simulink model "sampleModel26"  (Simulink 9.1)
settings: Solver=VariableStepAuto  StartTime=0.0  StopTime=10.0  RelTol=1e-3
undefined symbols (not defined in the file): DiscIntNeverNeededParam, Newton, Raphson
libraries: simulink x50
(part 1 of 2)
settings Model: Creator=DELL  LastModifiedBy=DELL
settings DataIOCC: SaveFormat=Dataset
settings OptimizationCC: LifeSpan=auto
settings DebuggingCC: UnderspecifiedInitializationDetection=Simplified  MergeDetectMultiDrivingBlocksExec=error  SFUnexpectedBacktrackingDiag=error  SFNoUnconditionalDefaultTransitionDiag=error  SFExecutionAtInitializationDiag=warning
settings HardwareCC: ProdBitPerPointer=64  ProdBitPerSizeT=64  ProdBitPerPtrDiffT=64  ProdLargestAtomicFloat=Float  ProdIntDivRoundTo=Zero  ProdEndianess=LittleEndian  ProdWordSize=64  ProdHWDeviceType=Intel->x86-64 (Windows64)
settings ModelReferenceCC: PropagateSignalLabelsOutOfModel=on
settings CodeAppCC: StateflowObjectComments=off
settings GRTTargetCC: TargetLangStandard=C99 (ISO)  CombineOutputUpdateFcns=on  GRTInterface=off
settings ConfigComp: CovMetricSettings=dwe  CovHtmlReporting=off  CovSaveCumulativeToWorkspaceVar=off  CovSaveSingleToWorkspaceVar=off  CovExternalEMLEnable=on

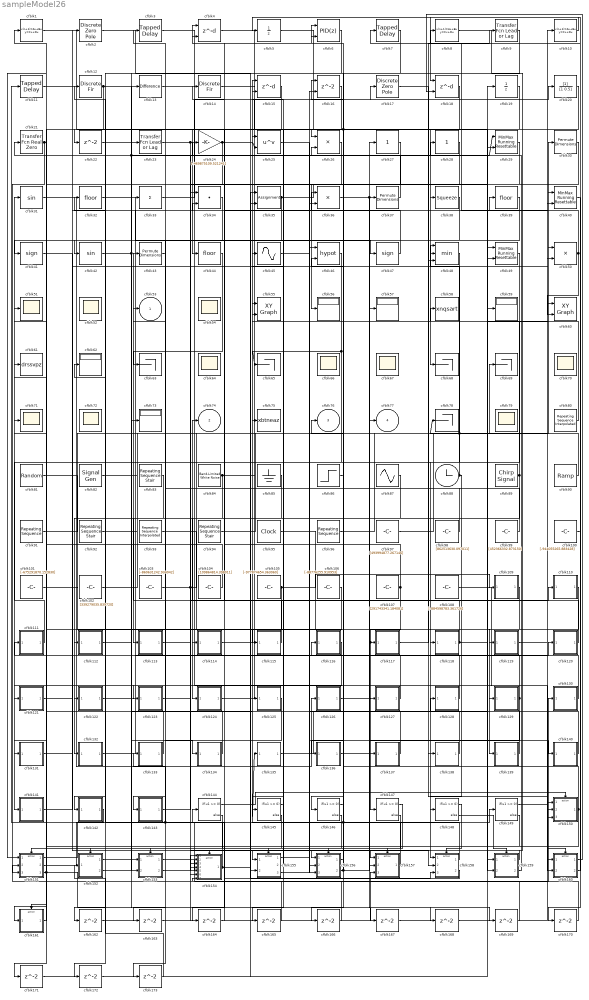
== system sampleModel26 ==
  cfblk1 : DiscreteStateSpace
  cfblk10 : DiscreteStateSpace
  cfblk100 : Constant  Value=[-944055265.883428]  SampleTime=1
  cfblk101 : Constant  Value=[-675291870.152830]  SampleTime=1
  cfblk102 : Constant  Value=[339279035.839720]  SampleTime=1
  cfblk103 : Constant  Value=[-860631242.934042]  SampleTime=1
  cfblk104 : Constant  Value=[109864814.398011]  SampleTime=1
  cfblk105 : Constant  Value=[-977874654.363060]  SampleTime=1
  cfblk106 : Constant  Value=[-88776255.910953]  SampleTime=1
  cfblk107 : Constant  Value=[291743341.184081]  SampleTime=1
  cfblk108 : Constant  Value=[-884598783.361726]  SampleTime=1
  cfblk109 : Subsystem
  cfblk11 : simulink/Discrete/Tapped Delay  vinit=0.0  samptime=-1  NumDelays=1  DelayOrder=Oldest  includeCurrent=off
  cfblk110 : Subsystem
  cfblk111 : Subsystem
  cfblk112 : Subsystem
  cfblk113 : Subsystem
  cfblk114 : Subsystem
  cfblk115 : Subsystem
  cfblk116 : Subsystem
  cfblk117 : Subsystem
  cfblk118 : Subsystem
  cfblk119 : Subsystem
  cfblk12 : DiscreteFir  SampleTime=1
  cfblk120 : Subsystem
  cfblk121 : Subsystem
  cfblk122 : Subsystem
  cfblk123 : Subsystem
  cfblk124 : Subsystem
  cfblk125 : Subsystem
  cfblk126 : Subsystem
  cfblk127 : Subsystem
  cfblk128 : Subsystem
  cfblk129 : Subsystem
  cfblk13 : simulink/Discrete/Difference  ICPrevInput=0.0  OutMin=[]  OutMax=[]  OutDataTypeStr=Inherit: Inherit via back propagation  OutDataType=fixdt(1, 16)  OutScaling=2^-10  DoSatur=off
  cfblk130 : Subsystem
  cfblk131 : Subsystem
  cfblk132 : Subsystem
  cfblk133 : Subsystem
  cfblk134 : Subsystem
  cfblk135 : Subsystem
  cfblk136 : Subsystem
  cfblk137 : Subsystem
  cfblk138 : Subsystem
  cfblk139 : Subsystem
  cfblk14 : DiscreteFir  SampleTime=1
  cfblk140 : Subsystem
  cfblk141 : Subsystem
  cfblk142 : Subsystem
  cfblk143 : Subsystem
  cfblk{144..149} (6 alike) : If  IfExpression=u1 >= 0  SampleTime=1
  cfblk15 : Delay  DelayLengthSource=Input port  SampleTime=1
      settings: InputPortMap=u0,p1
  cfblk150 : Subsystem  TreatAsAtomicUnit=on
  cfblk151 : Subsystem  TreatAsAtomicUnit=on
  cfblk152 : Subsystem  TreatAsAtomicUnit=on
  cfblk153 : Subsystem  TreatAsAtomicUnit=on
  cfblk154 : Subsystem  TreatAsAtomicUnit=on
  cfblk155 : Subsystem  TreatAsAtomicUnit=on
  cfblk156 : Subsystem  TreatAsAtomicUnit=on
  cfblk157 : Subsystem  TreatAsAtomicUnit=on
  cfblk158 : Subsystem  TreatAsAtomicUnit=on
  cfblk159 : Subsystem  TreatAsAtomicUnit=on
  cfblk16 : Delay  ShowEnablePort=on  SampleTime=1
      settings: InputPortMap=u0,e6
  cfblk160 : Subsystem  TreatAsAtomicUnit=on
  cfblk161 : Subsystem  TreatAsAtomicUnit=on
  cfblk{22,162..173} (13 alike) : Delay  SampleTime=1
  cfblk17 : DiscreteZeroPole  Poles=[0 0.5]  Gain=1
  cfblk18 : Delay  DelayLengthSource=Input port  SampleTime=1
      settings: InputPortMap=u0,p1
  cfblk19 : UnitDelay
  cfblk2 : DiscreteZeroPole  Poles=[0 0.5]  Gain=1
  cfblk20 : DiscreteFilter  SampleTime=1
  cfblk21 : simulink/Discrete/Transfer Fcn Real Zero  ZeroZ=0.75  ICPrevInput=0.0  DoSatur=off
      settings: SourceProductName=Simulink  SourceProductBaseCode=SL
  cfblk23 : simulink/Discrete/Transfer Fcn Lead or Lag  PoleZ=0.95  ZeroZ=0.75  ICPrevOutput=0.0  ICPrevInput=0.0  DoSatur=off
      settings: SourceProductName=Simulink  SourceProductBaseCode=SL
  cfblk24 : Gain  Gain=[-469875109.521241]
  cfblk25 : Math  Operator=pow  SaturateOnIntegerOverflow=on
  cfblk26 : Product  Inputs=**
  cfblk27 : simulink/Math Operations/Slider Gain  gain=1  low=0  high=2
  cfblk28 : simulink/Math Operations/Slider Gain  gain=1  low=0  high=2
  cfblk29 : simulink/Math Operations/MinMax Running Resettable  Function=min  vinit=0.0
  cfblk3 : simulink/Discrete/Tapped Delay  vinit=0.0  samptime=-1  NumDelays=1  DelayOrder=Oldest  includeCurrent=off
  cfblk30 : PermuteDimensions
  cfblk31 : Trigonometry
  cfblk32 : Rounding
  cfblk33 : Sum  Inputs=+
  cfblk34 : DotProduct  InputSameDT=on  OutDataTypeStr=Inherit: Inherit via internal rule
  cfblk35 : Assignment  DiagnosticForDimensions=Warning  IndexOptions=Index vector (dialog)  Indices=1  OutputSizes=1
  cfblk36 : Product  Inputs=**
  cfblk37 : PermuteDimensions
  cfblk38 : Squeeze
  cfblk39 : Rounding
  cfblk4 : Delay  DelayLengthSource=Input port  SampleTime=1
      settings: InputPortMap=u0,p1
  cfblk40 : simulink/Math Operations/MinMax Running Resettable  Function=min  vinit=0.0
  cfblk41 : Signum
  cfblk42 : Trigonometry
  cfblk43 : PermuteDimensions
  cfblk44 : Rounding
  cfblk45 : Sin  TimeSource=Use external signal  SampleTime=0
  cfblk46 : Math  Operator=hypot  SaturateOnIntegerOverflow=on
  cfblk47 : Signum
  cfblk48 : MinMax  Inputs=3
  cfblk49 : simulink/Math Operations/MinMax Running Resettable  Function=min  vinit=0.0
  cfblk5 : UnitDelay
  cfblk50 : Product  Inputs=**
  cfblk{51..52,54,64,66..67,70..72,79} (10 alike) : Scope
      cfblk52 settings: Floating=on
      cfblk54 settings: Floating=on
      cfblk64 settings: Floating=on
      cfblk66 settings: Floating=on
      cfblk67 settings: Floating=on
      cfblk70 settings: Floating=on
      cfblk72 settings: Floating=on
      cfblk79 settings: Floating=on
  cfblk55 : simulink/Sinks/XY Graph  xmin=-1  xmax=1  ymin=-1  ymax=1  st=-1
  cfblk{56..57,59,62,73} (5 alike) : Display
  cfblk58 : ToWorkspace  VariableName=xnqsart  SaveFormat=Timeseries  SampleTime=-1
  cfblk6 : simulink/Continuous/PID Controller (2DOF)  Controller=PID  TimeDomain=Discrete-time  SampleTime=1  IntegratorMethod=Forward Euler  FilterMethod=Forward Euler  Form=Parallel  UseFilter=on  ControllerParametersSource=internal  P=1  I=1  D=0  N=100  b=1  c=1  InitialConditionSource=internal  InitialConditionForIntegrator=0  InitialConditionForFilter=0  ExternalReset=none  LimitOutput=off  UpperSaturationLimit=inf  LowerSaturationLimit=-inf  LinearizeAsGain=off  AntiWindupMode=none  Kb=1  TrackingMode=off  Kt=1  PParamMin=[]  PParamMax=[]  IParamMin=[]  IParamMax=[]  DParamMin=[]  DParamMax=[]  NParamMin=[]  NParamMax=[]  bParamMin=[]  bParamMax=[]  cParamMin=[]  cParamMax=[]  KbParamMin=[]  KbParamMax=[]  KtParamMin=[]  KtParamMax=[]  POutMin=[]  POutMax=[]  IOutMin=[]  IOutMax=[]  DOutMin=[]  DOutMax=[]  NOutMin=[]  NOutMax=[]  bOutMin=[]  bOutMax=[]  cOutMin=[]  cOutMax=[]  KbOutMin=[]  KbOutMax=[]  KtOutMin=[]  KtOutMax=[]  IntegratorOutMin=[]  IntegratorOutMax=[]  FilterOutMin=[]  FilterOutMax=[]  SumOutMin=[]  SumOutMax=[]  Sum1OutMin=[]  Sum1OutMax=[]  Sum2OutMin=[]  Sum2OutMax=[]  Sum3OutMin=[]  Sum3OutMax=[]  SumI1OutMin=[]  SumI1OutMax=[]  SumI2OutMin=[]  SumI2OutMax=[]  SumI3OutMin=[]  SumI3OutMax=[]  SumDOutMin=[]  SumDOutMax=[]  SaturationOutMin=[]  SaturationOutMax=[]  IntegratorContinuousStateAttributes=''  IntegratorStateMustResolveToSignalObject=off  IntegratorRTWStateStorageClass=Auto  FilterContinuousStateAttributes=''  FilterStateMustResolveToSignalObject=off  FilterRTWStateStorageClass=Auto  DifferentiatorICPrevScaledInput=0  DifferentiatorOutMin=[]  DifferentiatorOutMax=[]  FilterDiffOutCoefMin=[]  FilterDiffOutCoefMax=[]  SumDenOutMin=[]  SumDenOutMax=[]  SumNumOutMin=[]  SumNumOutMax=[]  ReciprocalOutMin=[]  ReciprocalOutMax=[]  DivideOutMin=[]  DivideOutMax=[]  TunerSelectOption=Transfer Function Based (PID Tuner App)
  cfblk60 : simulink/Sinks/XY Graph  xmin=-1  xmax=1  ymin=-1  ymax=1  st=-1
  cfblk61 : ToWorkspace  VariableName=drssvpz  SaveFormat=Timeseries  SampleTime=-1
  cfblk{63,65,68..69,78} (5 alike) : Terminator
  cfblk7 : simulink/Discrete/Tapped Delay  vinit=0.0  samptime=-1  NumDelays=1  DelayOrder=Oldest  includeCurrent=off
  cfblk75 : ToWorkspace  VariableName=xbtneaz  SaveFormat=Timeseries  SampleTime=-1
  cfblk8 : DiscreteStateSpace
  cfblk80 : simulink/Sources/Repeating Sequence Interpolated  OutValues=[-870086056.287552, 370773277.954319, 830488176.422611, 465742111.805598, 678569411.851133]  TimeValues=[0 0.1 0.5 0.6 1].'  LookUpMeth=Use Input Above  tsamp=0.01  OutMin=[]  OutMax=[]  OutDataTypeStr=double  OutputDataTypeScalingMode=double  OutDataType=fixdt(0,8)  OutScaling=2^-10
  cfblk81 : RandomNumber  Mean=[-78779.881234]  Variance=[71497.435581]  Seed=[976810598.000000]  SampleTime=0.1
  cfblk82 : SignalGenerator  WaveForm=sawtooth  Amplitude=[-817770877.646447]  Units=rad/sec
  cfblk83 : simulink/Sources/Repeating Sequence Stair  OutValues=[-901777578.723992, 88442323.013596]  tsamp=-1  OutMin=[]  OutMax=[]  OutDataTypeStr=double  OutputDataTypeScalingMode=double  OutDataType=fixdt(0,8)  ConRadixGroup=Best Precision: Vector-wise  OutScaling=2^-12
  cfblk84 : simulink/Sources/Band-Limited White Noise  Cov=[7948973946.375312]  Ts=0.1  seed=[5409314968.000000]
  cfblk85 : Ground
  cfblk86 : Step  Time=[11.000000]  Before=[-400151099.096636]  After=[190757747.705962]  SampleTime=0
  cfblk87 : Sin  Amplitude=[354659647.057073]  Bias=[193541944.936040]  SampleTime=0
  cfblk88 : Clock
  cfblk89 : simulink/Sources/Chirp Signal  f1=[-369850949.258945]  T=[760476368.947257]  f2=[936374467.184043]
  cfblk9 : simulink/Discrete/Transfer Fcn Lead or Lag  PoleZ=0.95  ZeroZ=0.75  ICPrevOutput=0.0  ICPrevInput=0.0  DoSatur=off
      settings: SourceProductName=Simulink  SourceProductBaseCode=SL
  cfblk90 : simulink/Sources/Ramp  slope=[8410.056745]  start=[18.258992]  InitialOutput=[-749225.159430]
  cfblk91 : simulink/Sources/Repeating Sequence  rep_seq_t=[0 2]  rep_seq_y=[-517814795.198206, -35255627.160542]
  cfblk92 : simulink/Sources/Repeating Sequence Stair  OutValues=[835863876.894369, -444784532.168246]  tsamp=-1  OutMin=[]  OutMax=[]  OutDataTypeStr=double  OutputDataTypeScalingMode=double  OutDataType=fixdt(0,8)  ConRadixGroup=Best Precision: Vector-wise  OutScaling=2^-12
  cfblk93 : simulink/Sources/Repeating Sequence Interpolated  OutValues=[267695016.754361, 181372896.852040, -130030541.622114, 663922758.389939, -764731192.298473]  TimeValues=[0 0.1 0.5 0.6 1].'  LookUpMeth=Use Input Nearest  tsamp=0.01  OutMin=[]  OutMax=[]  OutDataTypeStr=double  OutputDataTypeScalingMode=double  OutDataType=fixdt(0,8)  OutScaling=2^-10
  cfblk94 : simulink/Sources/Repeating Sequence Stair  OutValues=[-345371034.383514, -603859266.066574]  tsamp=-1  OutMin=[]  OutMax=[]  OutDataTypeStr=double  OutputDataTypeScalingMode=double  OutDataType=fixdt(0,8)  ConRadixGroup=Best Precision: Vector-wise  OutScaling=2^-12
  cfblk95 : DigitalClock
  cfblk96 : simulink/Sources/Repeating Sequence  rep_seq_t=[0 2]  rep_seq_y=[617464177.285764, 681593510.401765]
  cfblk97 : Constant  Value=[493994877.267146]  SampleTime=1
  cfblk98 : Constant  Value=[862513630.097011]  SampleTime=1
  cfblk99 : Constant  Value=[452366332.873150]  SampleTime=1
  cfblk53 : Outport
  cfblk74 : Outport  Port=2
  cfblk76 : Outport  Port=3
  cfblk77 : Outport  Port=4
  wires:
  cfblk132/1(cfblk2) -> cfblk39/1
  cfblk4/1 -> cfblk26/1
  cfblk115/1(cfblk2) -> cfblk43/1
  cfblk8/1 -> cfblk156/1(cfblk1)
  cfblk31/1 -> cfblk126/1(cfblk1)
  cfblk124/1(cfblk2) -> cfblk20/1
  cfblk48/1 -> cfblk158/1(cfblk1)
  cfblk114/1(cfblk2) -> cfblk118/1(cfblk1)
  cfblk158/1(cfblk2) -> cfblk15/1
  cfblk97/1 -> cfblk30/1
  cfblk116/1(cfblk2) -> cfblk141/1(cfblk1)
  cfblk82/1 -> cfblk69/1
  cfblk33/1 -> cfblk17/1
  cfblk84/1 -> cfblk124/1(cfblk1), cfblk40/2
  cfblk135/1(cfblk2) -> cfblk19/1
  cfblk142/1(cfblk2) -> cfblk11/1
  cfblk22/1 -> cfblk73/1
  cfblk85/1 -> cfblk132/1(cfblk1)
  cfblk12/1 -> cfblk22/1, cfblk169/1
  cfblk129/1(cfblk2) -> cfblk147/1, cfblk6/2
  cfblk6/1 -> cfblk112/1(cfblk1)
  cfblk158/2(cfblk15) -> cfblk142/1(cfblk1)
  cfblk153/1(cfblk2) -> cfblk130/1(cfblk1)
  cfblk151/1(cfblk2) -> cfblk13/1
  cfblk109/1(cfblk2) -> cfblk139/1(cfblk1)
  cfblk28/1 -> cfblk161/1(cfblk1)
  cfblk3/1 -> cfblk160/1(cfblk1)
  cfblk102/1 -> cfblk49/1
  cfblk91/1 -> cfblk75/1
  cfblk27/1 -> cfblk56/1
  cfblk139/1(cfblk2) -> cfblk26/2
  cfblk49/1 -> cfblk121/1(cfblk1)
  cfblk37/1 -> cfblk25/1
  cfblk151/2(cfblk15) -> cfblk37/1
  cfblk13/1 -> cfblk160/2(cfblk15)
  cfblk15/1 -> cfblk44/1
  cfblk39/1 -> cfblk114/1(cfblk1)
  cfblk99/1 -> cfblk53/1
  cfblk103/1 -> cfblk34/1, cfblk48/3
  cfblk18/1 -> cfblk136/1(cfblk1), cfblk165/1
  cfblk95/1 -> cfblk129/1(cfblk1)
  cfblk93/1 -> cfblk159/1(cfblk1)
  cfblk14/1 -> cfblk68/1
  cfblk113/1(cfblk2) -> cfblk157/1(cfblk1)
  cfblk153/2(cfblk8) -> cfblk57/1
  cfblk21/1 -> cfblk151/1(cfblk1), cfblk151/3(cfblk14)
  cfblk111/1(cfblk2) -> cfblk31/1
  cfblk42/1 -> cfblk23/1, cfblk29/1, cfblk134/1(cfblk1)
  cfblk100/1 -> cfblk18/1
  cfblk87/1 -> cfblk113/1(cfblk1)
  cfblk50/1 -> cfblk8/1, cfblk60/2
  cfblk161/1(cfblk2) -> cfblk71/1
  cfblk119/1(cfblk2) -> cfblk10/1
  cfblk133/1(cfblk2) -> cfblk111/1(cfblk1)
  cfblk23/1 -> cfblk59/1, cfblk36/2
  cfblk143/1(cfblk2) -> cfblk28/1
  cfblk16/1 -> cfblk155/1(cfblk1)
  cfblk44/1 -> cfblk63/1
  cfblk126/1(cfblk2) -> cfblk137/1(cfblk1)
  cfblk131/1(cfblk2) -> cfblk34/2
  cfblk86/1 -> cfblk146/1
  cfblk2/1 -> cfblk155/2(cfblk11)
  cfblk26/1 -> cfblk115/1(cfblk1)
  cfblk92/1 -> cfblk46/1
  cfblk83/1 -> cfblk122/1(cfblk1)
  cfblk134/1(cfblk2) -> cfblk32/1
  cfblk160/1(cfblk2) -> cfblk18/2
  cfblk20/1 -> cfblk41/1
  cfblk157/1(cfblk2) -> cfblk135/1(cfblk1), cfblk76/1
  cfblk121/1(cfblk2) -> cfblk48/1
  cfblk35/1 -> cfblk38/1, cfblk172/1
  cfblk88/1 -> cfblk148/1, cfblk55/2
  cfblk138/1(cfblk2) -> cfblk116/1(cfblk1)
  cfblk101/1 -> cfblk157/2(cfblk16)
  cfblk106/1 -> cfblk145/1
  cfblk90/1 -> cfblk78/1, cfblk48/2
  cfblk122/1(cfblk2) -> cfblk120/1(cfblk1)
  cfblk112/1(cfblk2) -> cfblk153/1(cfblk1)
  cfblk24/1 -> cfblk25/2, cfblk154/5(cfblk15)
  cfblk130/1(cfblk2) -> cfblk15/2
  cfblk10/1 -> cfblk5/1
  cfblk29/1 -> cfblk35/2
  cfblk120/1(cfblk2) -> cfblk24/1
  cfblk1/1 -> cfblk138/1(cfblk1)
  cfblk5/1 -> cfblk159/2(cfblk9)
  cfblk25/1 -> cfblk140/1(cfblk1)
  cfblk9/1 -> cfblk153/2(cfblk7)
  cfblk136/1(cfblk2) -> cfblk77/1
  cfblk128/1(cfblk2) -> cfblk6/1
  cfblk108/1 -> cfblk150/1(cfblk1)
  cfblk150/1(cfblk2) -> cfblk36/1, cfblk163/1
  cfblk89/1 -> cfblk156/2(cfblk13), cfblk55/1
  cfblk110/1(cfblk2) -> cfblk119/1(cfblk1)
  cfblk32/1 -> cfblk47/1
  cfblk105/1 -> cfblk109/1(cfblk1), cfblk131/1(cfblk1)
  cfblk11/1 -> cfblk33/1
  cfblk34/1 -> cfblk123/1(cfblk1)
  cfblk17/1 -> cfblk150/2(cfblk10)
  cfblk36/1 -> cfblk27/1, cfblk168/1
  cfblk160/2(cfblk16) -> cfblk7/1
  cfblk30/1 -> cfblk42/1
  cfblk47/1 -> cfblk14/1
  cfblk45/1 -> cfblk156/3(cfblk14)
  cfblk156/1(cfblk2) -> cfblk46/2
  cfblk155/1(cfblk2) -> cfblk50/1
  cfblk118/1(cfblk2) -> cfblk74/1, cfblk60/1
  cfblk156/2(cfblk15) -> cfblk4/1, cfblk40/1
  cfblk151/3(cfblk16) -> cfblk61/1, cfblk167/1
  cfblk137/1(cfblk2) -> cfblk62/1
  cfblk41/1 -> cfblk158/2(cfblk13)
  cfblk81/1 -> cfblk154/2(cfblk12)
  cfblk98/1 -> cfblk16/1
  cfblk104/1 -> cfblk1/1
  cfblk80/1 -> cfblk58/1
  cfblk43/1 -> cfblk143/1(cfblk1)
  cfblk152/1(cfblk2) -> cfblk125/1(cfblk1)
  cfblk140/1(cfblk2) -> cfblk3/1
  cfblk141/1(cfblk2) -> cfblk2/1
  cfblk127/1(cfblk2) -> cfblk51/1
  cfblk94/1 -> cfblk16/2
  cfblk154/1(cfblk2) -> cfblk133/1(cfblk1), cfblk12/1, cfblk158/3(cfblk14)
  cfblk107/1 -> cfblk127/1(cfblk1), cfblk117/1(cfblk1), cfblk4/2
  cfblk96/1 -> cfblk49/2
  cfblk46/1 -> cfblk65/1, cfblk162/1
  cfblk152/2(cfblk9) -> cfblk149/1
  cfblk123/1(cfblk2) -> cfblk110/1(cfblk1)
  cfblk155/2(cfblk12) -> cfblk45/1
  cfblk117/1(cfblk2) -> cfblk9/1
  cfblk155/3(cfblk13) -> cfblk128/1(cfblk1)
  cfblk159/1(cfblk2) -> cfblk154/3(cfblk13)
  cfblk159/2(cfblk10) -> cfblk21/1
  cfblk144/1 -> cfblk150/Action
  cfblk144/2 -> cfblk151/Action
  cfblk145/1 -> cfblk152/Action
  cfblk145/2 -> cfblk153/Action
  cfblk146/1 -> cfblk154/Action
  cfblk146/2 -> cfblk155/Action
  cfblk147/1 -> cfblk156/Action
  cfblk147/2 -> cfblk157/Action
  cfblk148/1 -> cfblk158/Action
  cfblk148/2 -> cfblk159/Action
  cfblk149/1 -> cfblk160/Action
  cfblk149/2 -> cfblk161/Action
  cfblk162/1 -> cfblk154/6(cfblk16)
  cfblk163/1 -> cfblk157/3(cfblk17)
  cfblk19/1 -> cfblk164/1
  cfblk164/1 -> cfblk144/1
  cfblk165/1 -> cfblk154/7(cfblk17)
  cfblk7/1 -> cfblk166/1
  cfblk166/1 -> cfblk151/2(cfblk13)
  cfblk167/1 -> cfblk50/2
  cfblk168/1 -> cfblk150/3(cfblk11)
  cfblk169/1 -> cfblk154/4(cfblk14)
  cfblk40/1 -> cfblk170/1
  cfblk170/1 -> cfblk154/1(cfblk1)
  cfblk38/1 -> cfblk171/1
  cfblk171/1 -> cfblk35/1
  cfblk172/1 -> cfblk29/2
  cfblk125/1(cfblk2) -> cfblk173/1
  cfblk173/1 -> cfblk152/1(cfblk1)

== system sampleModel26/cfblk109 ==
  cfblk1 : Inport
  cfblk2 : Outport
  wires:
  cfblk1/1 -> cfblk2/1

== system sampleModel26/cfblk110 ==
  cfblk1 : Inport
  cfblk2 : Outport
  wires:
  cfblk1/1 -> cfblk2/1

== system sampleModel26/cfblk111 ==
  cfblk1 : Inport
  cfblk2 : Outport
  wires:
  cfblk1/1 -> cfblk2/1

== system sampleModel26/cfblk112 ==
  cfblk1 : Inport
  cfblk2 : Outport
  wires:
  cfblk1/1 -> cfblk2/1

== system sampleModel26/cfblk113 ==
  cfblk1 : Inport
  cfblk2 : Outport
  wires:
  cfblk1/1 -> cfblk2/1

== system sampleModel26/cfblk114 ==
  cfblk1 : Inport
  cfblk2 : Outport
  wires:
  cfblk1/1 -> cfblk2/1

== system sampleModel26/cfblk115 ==
  cfblk1 : Inport
  cfblk2 : Outport
  wires:
  cfblk1/1 -> cfblk2/1

== system sampleModel26/cfblk116 ==
  cfblk1 : Inport
  cfblk2 : Outport
  wires:
  cfblk1/1 -> cfblk2/1

== system sampleModel26/cfblk117 ==
  cfblk1 : Inport
  cfblk2 : Outport
  wires:
  cfblk1/1 -> cfblk2/1

== system sampleModel26/cfblk118 ==
  cfblk1 : Inport
  cfblk2 : Outport
  wires:
  cfblk1/1 -> cfblk2/1

== system sampleModel26/cfblk119 ==
  cfblk1 : Inport
  cfblk2 : Outport
  wires:
  cfblk1/1 -> cfblk2/1

== system sampleModel26/cfblk120 ==
  cfblk1 : Inport
  cfblk2 : Outport
  wires:
  cfblk1/1 -> cfblk2/1

== system sampleModel26/cfblk121 ==
  cfblk1 : Inport
  cfblk2 : Outport
  wires:
  cfblk1/1 -> cfblk2/1

== system sampleModel26/cfblk122 ==
  cfblk1 : Inport
  cfblk2 : Outport
  wires:
  cfblk1/1 -> cfblk2/1

== system sampleModel26/cfblk123 ==
  cfblk1 : Inport
  cfblk2 : Outport
  wires:
  cfblk1/1 -> cfblk2/1

== system sampleModel26/cfblk124 ==
  cfblk1 : Inport
  cfblk2 : Outport
  wires:
  cfblk1/1 -> cfblk2/1

== system sampleModel26/cfblk125 ==
  cfblk1 : Inport
  cfblk2 : Outport
  wires:
  cfblk1/1 -> cfblk2/1

== system sampleModel26/cfblk126 ==
  cfblk1 : Inport
  cfblk2 : Outport
  wires:
  cfblk1/1 -> cfblk2/1

== system sampleModel26/cfblk127 ==
  cfblk1 : Inport
  cfblk2 : Outport
  wires:
  cfblk1/1 -> cfblk2/1

== system sampleModel26/cfblk128 ==
  cfblk1 : Inport
  cfblk2 : Outport
  wires:
  cfblk1/1 -> cfblk2/1

== system sampleModel26/cfblk129 ==
  cfblk1 : Inport
  cfblk2 : Outport
  wires:
  cfblk1/1 -> cfblk2/1

== system sampleModel26/cfblk130 ==
  cfblk1 : Inport
  cfblk2 : Outport
  wires:
  cfblk1/1 -> cfblk2/1

== system sampleModel26/cfblk131 ==
  cfblk1 : Inport
  cfblk2 : Outport
  wires:
  cfblk1/1 -> cfblk2/1

== system sampleModel26/cfblk132 ==
  cfblk1 : Inport
  cfblk2 : Outport
  wires:
  cfblk1/1 -> cfblk2/1

== system sampleModel26/cfblk133 ==
  cfblk1 : Inport
  cfblk2 : Outport
  wires:
  cfblk1/1 -> cfblk2/1

== system sampleModel26/cfblk134 ==
  cfblk1 : Inport
  cfblk2 : Outport
  wires:
  cfblk1/1 -> cfblk2/1

== system sampleModel26/cfblk135 ==
  cfblk1 : Inport
  cfblk2 : Outport
  wires:
  cfblk1/1 -> cfblk2/1

== system sampleModel26/cfblk136 ==
  cfblk1 : Inport
  cfblk2 : Outport
  wires:
  cfblk1/1 -> cfblk2/1

== system sampleModel26/cfblk137 ==
  cfblk1 : Inport
  cfblk2 : Outport
  wires:
  cfblk1/1 -> cfblk2/1

== system sampleModel26/cfblk138 ==
  cfblk1 : Inport
  cfblk2 : Outport
  wires:
  cfblk1/1 -> cfblk2/1

== system sampleModel26/cfblk139 ==
  cfblk1 : Inport
  cfblk2 : Outport
  wires:
  cfblk1/1 -> cfblk2/1

== system sampleModel26/cfblk140 ==
  cfblk1 : Inport
  cfblk2 : Outport
  wires:
  cfblk1/1 -> cfblk2/1

== system sampleModel26/cfblk141 ==
  cfblk1 : Inport
  cfblk2 : Outport
  wires:
  cfblk1/1 -> cfblk2/1

== system sampleModel26/cfblk142 ==
  cfblk1 : Inport
  cfblk2 : Outport
  wires:
  cfblk1/1 -> cfblk2/1

== system sampleModel26/cfblk143 ==
  cfblk1 : Inport
  cfblk2 : Outport
  wires:
  cfblk1/1 -> cfblk2/1

== system sampleModel26/cfblk150 ==
  cfblk1 : Inport
  cfblk10 : Inport  Port=2
  cfblk11 : Inport  Port=3
  Action Port : ActionPort  ActionType=then
  cfblk12 : Delay
  cfblk3 : simulink/Discrete/Tapped Delay  vinit=0.0  samptime=-1  NumDelays=1  DelayOrder=Oldest  includeCurrent=off
  cfblk4 : MinMax  Function=max  Inputs=3
  cfblk5 : Polyval  Coefs=[ +2.081618890e-019, -1.441693666e-014, +4.719686976e-010, -8.536869453e-006, +1.621573104e-001, -8.087801117e+001 ]
  cfblk6 : Product
  cfblk7 : Product  Inputs=*
  cfblk8 : Subsystem
  cfblk9 : Subsystem
  cfblk2 : Outport
  wires:
  cfblk1/1 -> cfblk6/1
  cfblk11/1 -> cfblk2/1, cfblk4/3
  cfblk8/1(cfblk2) -> cfblk5/1
  cfblk9/1(cfblk2) -> cfblk3/1
  cfblk5/1 -> cfblk4/1
  cfblk10/1 -> cfblk7/1
  cfblk6/1 -> cfblk8/1(cfblk1)
  cfblk7/1 -> cfblk6/2
  cfblk4/1 -> cfblk9/1(cfblk1)
  cfblk3/1 -> cfblk12/1
  cfblk12/1 -> cfblk4/2

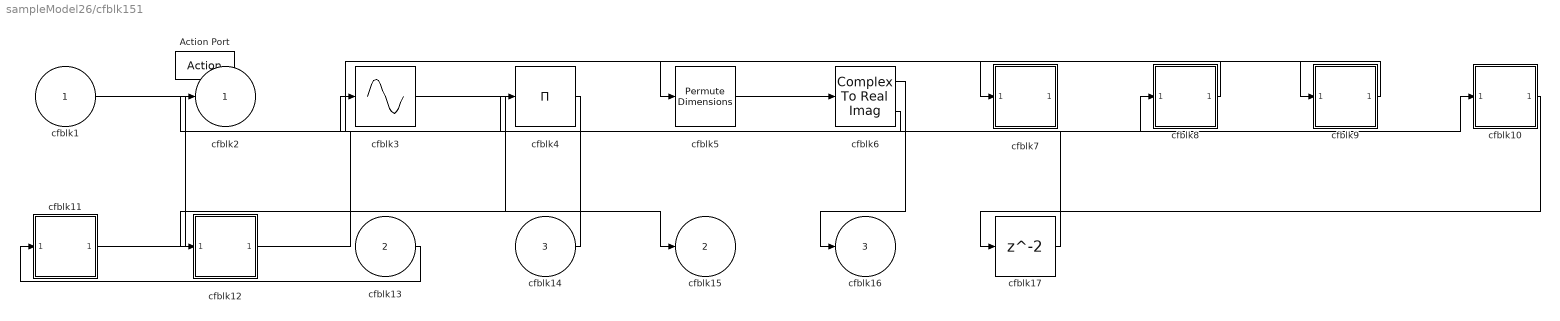
== system sampleModel26/cfblk151 ==
  cfblk1 : Inport
  cfblk13 : Inport  Port=2
  cfblk14 : Inport  Port=3
  Action Port : ActionPort  ActionType=else
  cfblk10 : Subsystem
  cfblk11 : Subsystem
  cfblk12 : Subsystem
  cfblk17 : Delay
  cfblk3 : Sin  TimeSource=Use external signal  SampleTime=0
  cfblk4 : Product  Inputs=*
  cfblk5 : PermuteDimensions
  cfblk6 : ComplexToRealImag
  cfblk7 : Subsystem
  cfblk8 : Subsystem
  cfblk9 : Subsystem
  cfblk2 : Outport
  cfblk15 : Outport  Port=2
  cfblk16 : Outport  Port=3
  wires:
  cfblk12/1(cfblk2) -> cfblk10/1(cfblk1)
  cfblk11/1(cfblk2) -> cfblk9/1(cfblk1)
  cfblk5/1 -> cfblk6/1
  cfblk1/1 -> cfblk8/1(cfblk1)
  cfblk3/1 -> cfblk15/1
  cfblk9/1(cfblk2) -> cfblk7/1(cfblk1)
  cfblk6/1 -> cfblk16/1
  cfblk14/1 -> cfblk3/1
  cfblk4/1 -> cfblk12/1(cfblk1)
  cfblk13/1 -> cfblk11/1(cfblk1)
  cfblk8/1(cfblk2) -> cfblk5/1
  cfblk6/2 -> cfblk2/1
  cfblk10/1(cfblk2) -> cfblk17/1
  cfblk17/1 -> cfblk4/1

== system sampleModel26/cfblk152 ==
  cfblk1 : Inport
  Action Port : ActionPort  ActionType=then
  cfblk10 : Delay
  cfblk3 : DiscreteTransferFcn
  cfblk4 : Sum  Inputs=+-
  cfblk5 : Abs
  cfblk6 : Bias  Bias=[-166739738.922034]
  cfblk7 : Sqrt  SaturateOnIntegerOverflow=on
  cfblk8 : Subsystem
  cfblk2 : Outport
  cfblk9 : Outport  Port=2
  wires:
  cfblk6/1 -> cfblk9/1
  cfblk8/1(cfblk2) -> cfblk4/1, cfblk5/1
  cfblk3/1 -> cfblk7/1
  cfblk7/1 -> cfblk8/1(cfblk1)
  cfblk5/1 -> cfblk4/2
  cfblk4/1 -> cfblk6/1, cfblk10/1
  cfblk1/1 -> cfblk2/1
  cfblk10/1 -> cfblk3/1

== system sampleModel26/cfblk153 ==
  cfblk1 : Inport
  cfblk7 : Inport  Port=2
  Action Port : ActionPort  ActionType=else
  cfblk3 : simulink/Math Operations/Slider Gain  gain=1  low=0  high=2
  cfblk4 : Product
  cfblk5 : Product  Inputs=*
  cfblk6 : Subsystem
  cfblk2 : Outport
  cfblk8 : Outport  Port=2
  wires:
  cfblk3/1 -> cfblk8/1
  cfblk7/1 -> cfblk6/1(cfblk1)
  cfblk5/1 -> cfblk4/1, cfblk3/1
  cfblk4/1 -> cfblk2/1
  cfblk6/1(cfblk2) -> cfblk5/1
  cfblk1/1 -> cfblk4/2

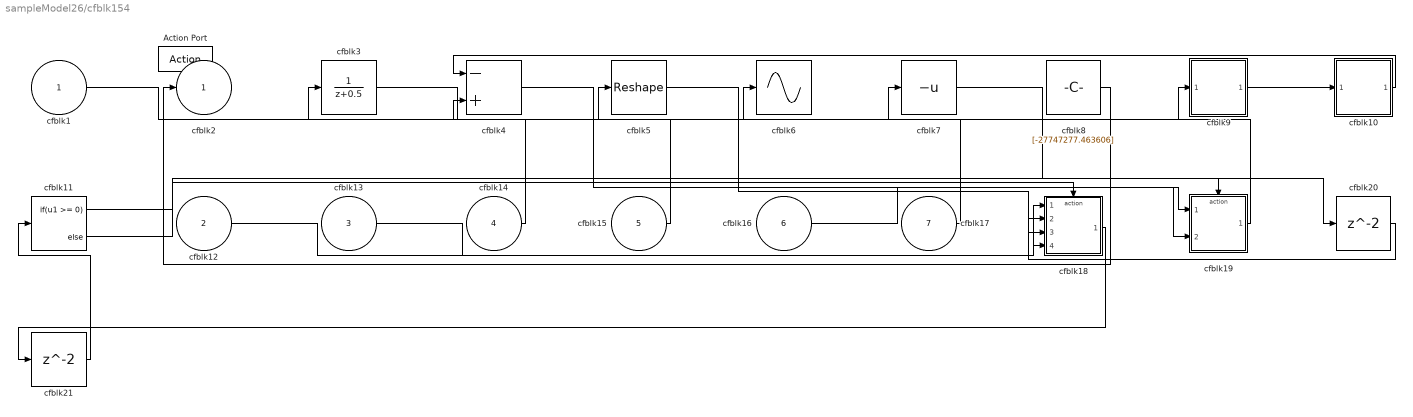
== system sampleModel26/cfblk154 ==
  cfblk1 : Inport
  cfblk12 : Inport  Port=2
  cfblk13 : Inport  Port=3
  cfblk14 : Inport  Port=4
  cfblk15 : Inport  Port=5
  cfblk16 : Inport  Port=6
  cfblk17 : Inport  Port=7
  Action Port : ActionPort  ActionType=then
  cfblk10 : Subsystem
  cfblk11 : If  IfExpression=u1 >= 0  SampleTime=1
  cfblk18 : Subsystem  TreatAsAtomicUnit=on
  cfblk19 : Subsystem  TreatAsAtomicUnit=on
  cfblk20 : Delay
  cfblk21 : Delay
  cfblk3 : DiscreteTransferFcn
  cfblk4 : Sum  Inputs=-+
  cfblk5 : Reshape
  cfblk6 : Sin  TimeSource=Use external signal  SampleTime=0
  cfblk7 : UnaryMinus
  cfblk8 : Constant  Value=[-27747277.463606]  SampleTime=1
  cfblk9 : Subsystem
  cfblk2 : Outport
  wires:
  cfblk14/1 -> cfblk3/1
  cfblk12/1 -> cfblk18/1(cfblk1)
  cfblk10/1(cfblk2) -> cfblk4/1
  cfblk9/1(cfblk2) -> cfblk10/1(cfblk1)
  cfblk3/1 -> cfblk6/1
  cfblk5/1 -> cfblk18/3(cfblk15)
  cfblk8/1 -> cfblk2/1
  cfblk17/1 -> cfblk5/1
  cfblk15/1 -> cfblk4/2
  cfblk13/1 -> cfblk18/4(cfblk16)
  cfblk16/1 -> cfblk19/1(cfblk1)
  cfblk4/1 -> cfblk19/2(cfblk9)
  cfblk19/1(cfblk2) -> cfblk7/1
  cfblk1/1 -> cfblk9/1(cfblk1)
  cfblk11/1 -> cfblk18/Action
  cfblk11/2 -> cfblk19/Action
  cfblk7/1 -> cfblk20/1
  cfblk20/1 -> cfblk18/2(cfblk14)
  cfblk18/1(cfblk2) -> cfblk21/1
  cfblk21/1 -> cfblk11/1

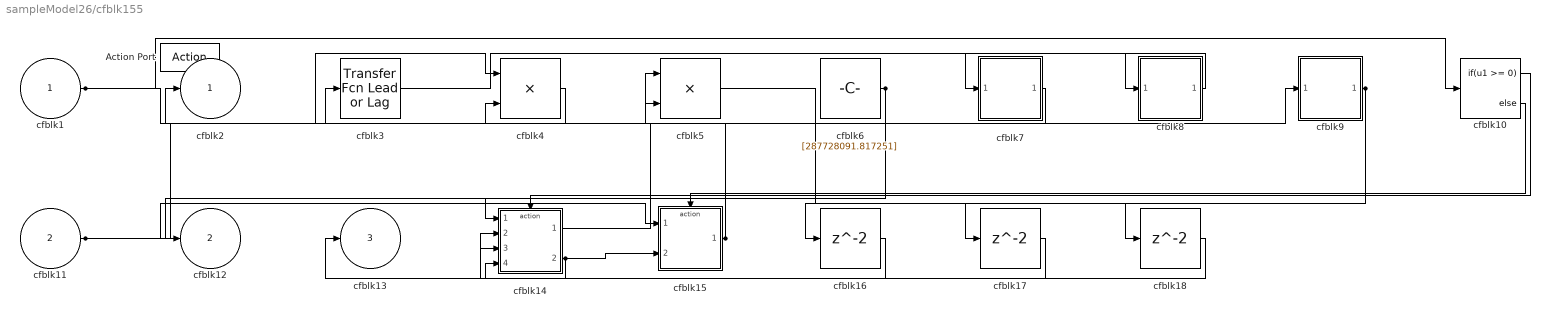
== system sampleModel26/cfblk155 ==
  cfblk1 : Inport
  cfblk11 : Inport  Port=2
  Action Port : ActionPort  ActionType=else
  cfblk10 : If  IfExpression=u1 >= 0  SampleTime=1
  cfblk14 : Subsystem  TreatAsAtomicUnit=on
  cfblk15 : Subsystem  TreatAsAtomicUnit=on
  cfblk16 : Delay
  cfblk17 : Delay
  cfblk18 : Delay
  cfblk3 : simulink/Discrete/Transfer Fcn Lead or Lag  PoleZ=0.95  ZeroZ=0.75  ICPrevOutput=0.0  ICPrevInput=0.0  DoSatur=off
      settings: SourceProductName=Simulink  SourceProductBaseCode=SL
  cfblk4 : Product  Inputs=**
  cfblk5 : Product  Inputs=**
  cfblk6 : Constant  Value=[287728091.817251]  SampleTime=1
  cfblk7 : Subsystem
  cfblk8 : Subsystem
  cfblk9 : Subsystem
  cfblk2 : Outport
  cfblk12 : Outport  Port=2
  cfblk13 : Outport  Port=3
  wires:
  cfblk3/1 -> cfblk8/1(cfblk1)
  cfblk14/1(cfblk2) -> cfblk9/1(cfblk1)
  cfblk15/1(cfblk2) -> cfblk5/1, cfblk4/2
  cfblk1/1 -> cfblk10/1, cfblk5/2
  cfblk4/1 -> cfblk3/1
  cfblk6/1 -> cfblk14/1(cfblk1), cfblk12/1
  cfblk8/1(cfblk2) -> cfblk7/1(cfblk1)
  cfblk11/1 -> cfblk4/1, cfblk15/1(cfblk1)
  cfblk9/1(cfblk2) -> cfblk16/1, cfblk17/1
  cfblk14/2(cfblk17) -> cfblk13/1, cfblk15/2(cfblk8)
  cfblk7/1(cfblk2) -> cfblk2/1
  cfblk10/1 -> cfblk14/Action
  cfblk10/2 -> cfblk15/Action
  cfblk16/1 -> cfblk14/3(cfblk15)
  cfblk17/1 -> cfblk14/4(cfblk16)
  cfblk5/1 -> cfblk18/1
  cfblk18/1 -> cfblk14/2(cfblk14)

== system sampleModel26/cfblk156 ==
  cfblk1 : Inport
  cfblk13 : Inport  Port=2
  cfblk14 : Inport  Port=3
  Action Port : ActionPort  ActionType=then
  cfblk10 : Subsystem
  cfblk11 : Subsystem
  cfblk12 : Subsystem
  cfblk3 : DiscreteZeroPole  Poles=[0 0.5]  Gain=1  SampleTime=-1
  cfblk4 : Polyval  Coefs=[ +2.081618890e-019, -1.441693666e-014, +4.719686976e-010, -8.536869453e-006, +1.621573104e-001, -8.087801117e+001 ]
  cfblk5 : Rounding
  cfblk6 : Polyval  Coefs=[ +2.081618890e-019, -1.441693666e-014, +4.719686976e-010, -8.536869453e-006, +1.621573104e-001, -8.087801117e+001 ]
  cfblk7 : Constant  Value=[-425518859.067546]  SampleTime=1
  cfblk8 : Subsystem
  cfblk9 : Subsystem
  cfblk2 : Outport
  cfblk15 : Outport  Port=2
  wires:
  cfblk1/1 -> cfblk5/1
  cfblk6/1 -> cfblk4/1
  cfblk12/1(cfblk2) -> cfblk3/1
  cfblk7/1 -> cfblk6/1
  cfblk10/1(cfblk2) -> cfblk8/1(cfblk1)
  cfblk4/1 -> cfblk11/1(cfblk1)
  cfblk13/1 -> cfblk2/1
  cfblk9/1(cfblk2) -> cfblk10/1(cfblk1)
  cfblk14/1 -> cfblk12/1(cfblk1)
  cfblk8/1(cfblk2) -> cfblk15/1
  cfblk11/1(cfblk2) -> cfblk9/1(cfblk1)

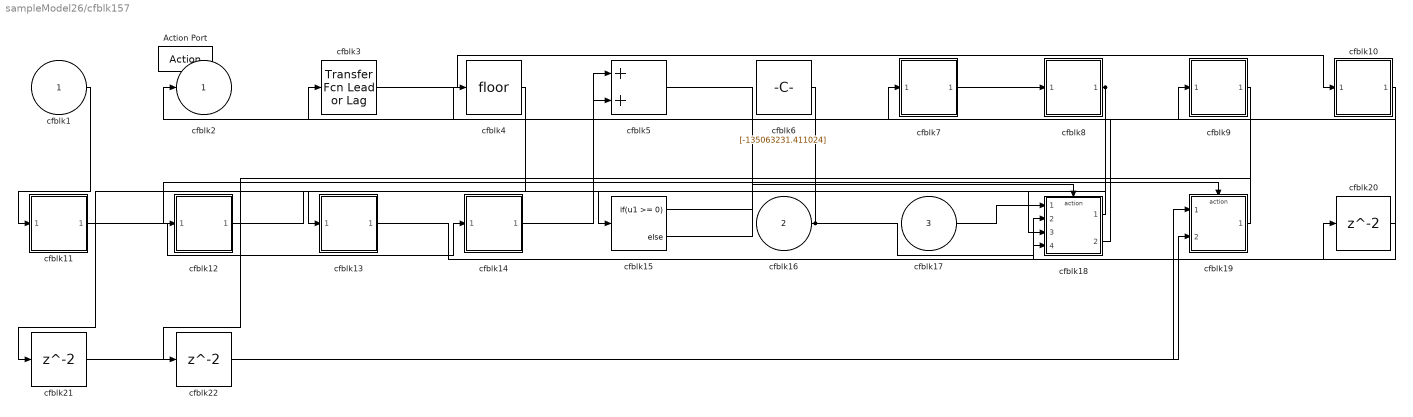
== system sampleModel26/cfblk157 ==
  cfblk1 : Inport
  cfblk16 : Inport  Port=2
  cfblk17 : Inport  Port=3
  Action Port : ActionPort  ActionType=else
  cfblk10 : Subsystem
  cfblk11 : Subsystem
  cfblk12 : Subsystem
  cfblk13 : Subsystem
  cfblk14 : Subsystem
  cfblk15 : If  IfExpression=u1 >= 0  SampleTime=1
  cfblk18 : Subsystem  TreatAsAtomicUnit=on
  cfblk19 : Subsystem  TreatAsAtomicUnit=on
  cfblk20 : Delay
  cfblk21 : Delay
  cfblk22 : Delay
  cfblk3 : simulink/Discrete/Transfer Fcn Lead or Lag  PoleZ=0.95  ZeroZ=0.75  ICPrevOutput=0.0  ICPrevInput=0.0  DoSatur=off
      settings: SourceProductName=Simulink  SourceProductBaseCode=SL
  cfblk4 : Rounding
  cfblk5 : Sum
  cfblk6 : Constant  Value=[-135063231.411024]  SampleTime=1
  cfblk7 : Subsystem
  cfblk8 : Subsystem
  cfblk9 : Subsystem
  cfblk2 : Outport
  wires:
  cfblk8/1(cfblk2) -> cfblk13/1(cfblk1), cfblk2/1
  cfblk7/1(cfblk2) -> cfblk8/1(cfblk1)
  cfblk11/1(cfblk2) -> cfblk14/1(cfblk1)
  cfblk3/1 -> cfblk10/1(cfblk1)
  cfblk6/1 -> cfblk12/1(cfblk1)
  cfblk12/1(cfblk2) -> cfblk15/1
  cfblk17/1 -> cfblk18/1(cfblk1)
  cfblk19/1(cfblk2) -> cfblk9/1(cfblk1)
  cfblk10/1(cfblk2) -> cfblk18/2(cfblk8)
  cfblk18/1(cfblk2) -> cfblk7/1(cfblk1)
  cfblk18/2(cfblk11) -> cfblk4/1
  cfblk1/1 -> cfblk11/1(cfblk1)
  cfblk5/1 -> cfblk18/3(cfblk9)
  cfblk16/1 -> cfblk3/1, cfblk18/4(cfblk10)
  cfblk14/1(cfblk2) -> cfblk5/2
  cfblk15/1 -> cfblk18/Action
  cfblk15/2 -> cfblk19/Action
  cfblk13/1(cfblk2) -> cfblk20/1
  cfblk20/1 -> cfblk5/1
  cfblk4/1 -> cfblk21/1
  cfblk21/1 -> cfblk19/1(cfblk1)
  cfblk9/1(cfblk2) -> cfblk22/1
  cfblk22/1 -> cfblk19/2(cfblk7)

== system sampleModel26/cfblk158 ==
  cfblk1 : Inport
  cfblk13 : Inport  Port=2
  cfblk14 : Inport  Port=3
  Action Port : ActionPort  ActionType=then
  cfblk10 : Constant  Value=[354864069.399818]  SampleTime=1
  cfblk11 : Subsystem
  cfblk12 : Subsystem
  cfblk16 : Delay
  cfblk3 : simulink/Discrete/Transfer Fcn Real Zero  ZeroZ=0.75  ICPrevInput=0.0  DoSatur=off
      settings: SourceProductName=Simulink  SourceProductBaseCode=SL
  cfblk4 : DiscreteStateSpace  SampleTime=-1
  cfblk5 : DiscreteTransferFcn
  cfblk6 : DiscreteIntegrator  SampleTime=-1  ICPrevOutput=DiscIntNeverNeededParam  ICPrevScaledInput=DiscIntNeverNeededParam
  cfblk7 : simulink/Math Operations/MinMax Running Resettable  Function=min  vinit=0.0
  cfblk8 : Sqrt  SaturateOnIntegerOverflow=on
  cfblk9 : Sum  Inputs=+
  cfblk2 : Outport
  cfblk15 : Outport  Port=2
  wires:
  cfblk4/1 -> cfblk6/1
  cfblk10/1 -> cfblk3/1
  cfblk1/1 -> cfblk4/1
  cfblk5/1 -> cfblk12/1(cfblk1)
  cfblk3/1 -> cfblk2/1
  cfblk14/1 -> cfblk11/1(cfblk1)
  cfblk11/1(cfblk2) -> cfblk5/1
  cfblk6/1 -> cfblk15/1
  cfblk13/1 -> cfblk7/1
  cfblk12/1(cfblk2) -> cfblk8/1
  cfblk7/1 -> cfblk9/1
  cfblk9/1 -> cfblk16/1
  cfblk16/1 -> cfblk7/2

== system sampleModel26/cfblk159 ==
  cfblk1 : Inport
  cfblk9 : Inport  Port=2
  Action Port : ActionPort  ActionType=else
  cfblk3 : simulink/Discrete/Transfer Fcn Real Zero  ZeroZ=0.75  ICPrevInput=0.0  DoSatur=off
      settings: SourceProductName=Simulink  SourceProductBaseCode=SL
  cfblk4 : UnitDelay  SampleTime=-1
  cfblk5 : Product  Inputs=*
  cfblk6 : Constant  Value=[-346399898.795938]  SampleTime=1
  cfblk7 : Subsystem
  cfblk8 : Subsystem
  cfblk2 : Outport
  cfblk10 : Outport  Port=2
  wires:
  cfblk8/1(cfblk2) -> cfblk5/1
  cfblk6/1 -> cfblk8/1(cfblk1)
  cfblk5/1 -> cfblk3/1
  cfblk3/1 -> cfblk7/1(cfblk1)
  cfblk7/1(cfblk2) -> cfblk10/1
  cfblk1/1 -> cfblk4/1
  cfblk4/1 -> cfblk2/1

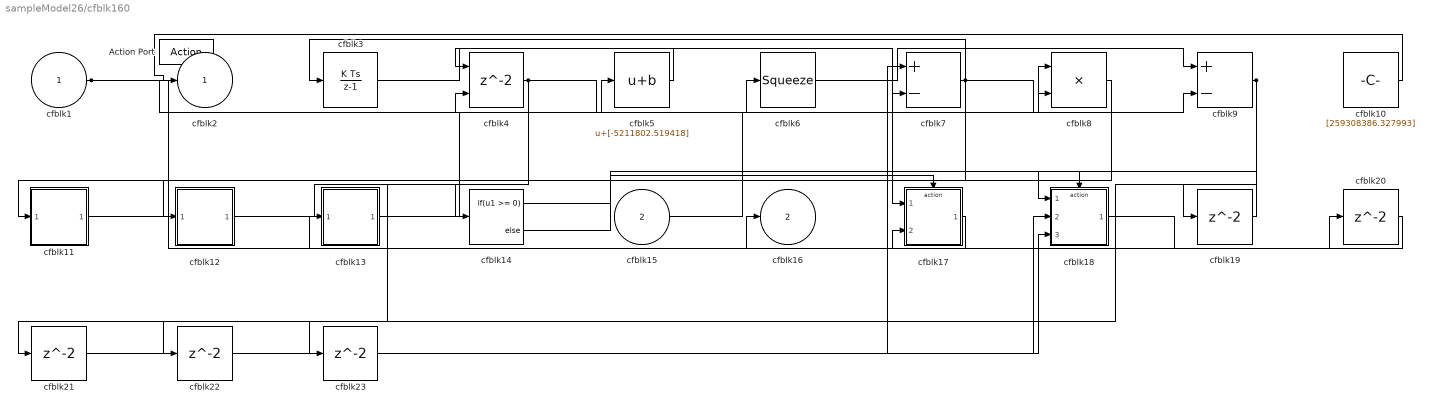
== system sampleModel26/cfblk160 ==
  cfblk1 : Inport
  cfblk15 : Inport  Port=2
  Action Port : ActionPort  ActionType=then
  cfblk10 : Constant  Value=[259308386.327993]  SampleTime=1
  cfblk11 : Subsystem
  cfblk12 : Subsystem
  cfblk13 : Subsystem
  cfblk14 : If  IfExpression=u1 >= 0  SampleTime=1
  cfblk17 : Subsystem  TreatAsAtomicUnit=on
  cfblk18 : Subsystem  TreatAsAtomicUnit=on
  cfblk{19..23} (5 alike) : Delay
  cfblk3 : DiscreteIntegrator  SampleTime=-1  ICPrevOutput=DiscIntNeverNeededParam  ICPrevScaledInput=DiscIntNeverNeededParam
  cfblk4 : Delay  ShowEnablePort=on
      settings: InputPortMap=u0,e6
  cfblk5 : Bias  Bias=[-5211802.519418]
  cfblk6 : Squeeze
  cfblk7 : Sum  Inputs=+-
  cfblk8 : Product  Inputs=**
  cfblk9 : Sum  Inputs=+-
  cfblk2 : Outport
  cfblk16 : Outport  Port=2
  wires:
  cfblk13/1(cfblk2) -> cfblk6/1
  cfblk1/1 -> cfblk16/1, cfblk7/2
  cfblk11/1(cfblk2) -> cfblk5/1
  cfblk12/1(cfblk2) -> cfblk14/1
  cfblk10/1 -> cfblk2/1
  cfblk3/1 -> cfblk17/1(cfblk1)
  cfblk7/1 -> cfblk3/1, cfblk4/2, cfblk11/1(cfblk1), cfblk9/2
  cfblk9/1 -> cfblk19/1, cfblk21/1, cfblk22/1
  cfblk8/1 -> cfblk12/1(cfblk1)
  cfblk6/1 -> cfblk9/1
  cfblk5/1 -> cfblk4/1
  cfblk17/1(cfblk2) -> cfblk13/1(cfblk1)
  cfblk4/1 -> cfblk8/2, cfblk23/1
  cfblk15/1 -> cfblk8/1
  cfblk14/1 -> cfblk17/Action
  cfblk14/2 -> cfblk18/Action
  cfblk19/1 -> cfblk18/1(cfblk1)
  cfblk18/1(cfblk2) -> cfblk20/1
  cfblk20/1 -> cfblk17/2(cfblk12)
  cfblk21/1 -> cfblk18/2(cfblk10)
  cfblk22/1 -> cfblk18/3(cfblk11)
  cfblk23/1 -> cfblk7/1

== system sampleModel26/cfblk161 ==
  cfblk1 : Inport
  Action Port : ActionPort  ActionType=else
  cfblk10 : Subsystem
  cfblk11 : Subsystem
  cfblk12 : Subsystem
  cfblk13 : Subsystem
  cfblk14 : Delay
  cfblk15 : Delay
  cfblk3 : DiscreteFir
  cfblk4 : Product  Inputs=**
  cfblk5 : Sum  Inputs=+-
  cfblk6 : Product  Inputs=**
  cfblk7 : Constant  Value=[-196636644.575386]  SampleTime=1
  cfblk8 : Subsystem
  cfblk9 : Subsystem
  cfblk2 : Outport
  wires:
  cfblk3/1 -> cfblk9/1(cfblk1), cfblk6/2
  cfblk13/1(cfblk2) -> cfblk8/1(cfblk1)
  cfblk12/1(cfblk2) -> cfblk11/1(cfblk1)
  cfblk9/1(cfblk2) -> cfblk2/1
  cfblk8/1(cfblk2) -> cfblk3/1
  cfblk7/1 -> cfblk4/1
  cfblk6/1 -> cfblk5/1
  cfblk1/1 -> cfblk13/1(cfblk1)
  cfblk4/1 -> cfblk14/1, cfblk15/1
  cfblk10/1(cfblk2) -> cfblk12/1(cfblk1)
  cfblk11/1(cfblk2) -> cfblk4/2
  cfblk5/1 -> cfblk10/1(cfblk1)
  cfblk14/1 -> cfblk6/1
  cfblk15/1 -> cfblk5/2

== system sampleModel26/cfblk150/cfblk8 ==
  cfblk1 : Inport
  cfblk2 : Outport
  wires:
  cfblk1/1 -> cfblk2/1

== system sampleModel26/cfblk150/cfblk9 ==
  cfblk1 : Inport
  cfblk2 : Outport
  wires:
  cfblk1/1 -> cfblk2/1

== system sampleModel26/cfblk151/cfblk10 ==
  cfblk1 : Inport
  cfblk2 : Outport
  wires:
  cfblk1/1 -> cfblk2/1

== system sampleModel26/cfblk151/cfblk11 ==
  cfblk1 : Inport
  cfblk2 : Outport
  wires:
  cfblk1/1 -> cfblk2/1

== system sampleModel26/cfblk151/cfblk12 ==
  cfblk1 : Inport
  cfblk2 : Outport
  wires:
  cfblk1/1 -> cfblk2/1

== system sampleModel26/cfblk151/cfblk7 ==
  cfblk1 : Inport
  cfblk2 : Outport
  wires:
  cfblk1/1 -> cfblk2/1

== system sampleModel26/cfblk151/cfblk8 ==
  cfblk1 : Inport
  cfblk2 : Outport
  wires:
  cfblk1/1 -> cfblk2/1

== system sampleModel26/cfblk151/cfblk9 ==
  cfblk1 : Inport
  cfblk2 : Outport
  wires:
  cfblk1/1 -> cfblk2/1

== system sampleModel26/cfblk152/cfblk8 ==
  cfblk1 : Inport
  cfblk2 : Outport
  wires:
  cfblk1/1 -> cfblk2/1

== system sampleModel26/cfblk153/cfblk6 ==
  cfblk1 : Inport
  cfblk2 : Outport
  wires:
  cfblk1/1 -> cfblk2/1

== system sampleModel26/cfblk154/cfblk10 ==
  cfblk1 : Inport
  cfblk2 : Outport
  wires:
  cfblk1/1 -> cfblk2/1

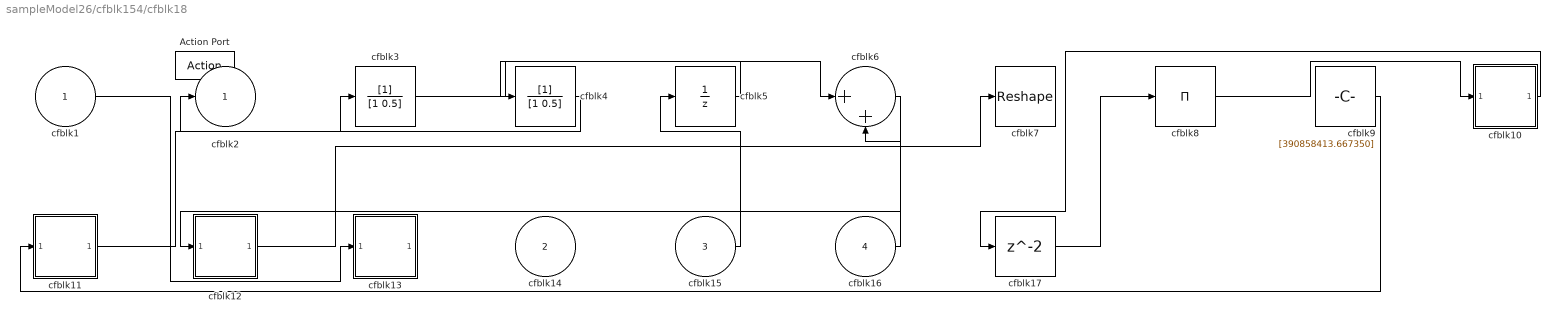
== system sampleModel26/cfblk154/cfblk18 ==
  cfblk1 : Inport
  cfblk14 : Inport  Port=2
  cfblk15 : Inport  Port=3
  cfblk16 : Inport  Port=4
  Action Port : ActionPort  ActionType=then
  cfblk10 : Subsystem
  cfblk11 : Subsystem
  cfblk12 : Subsystem
  cfblk13 : Subsystem
  cfblk17 : Delay
  cfblk3 : DiscreteFilter
  cfblk4 : DiscreteFilter
  cfblk5 : UnitDelay  SampleTime=-1
  cfblk6 : Sum  Inputs=|++
  cfblk7 : Reshape
  cfblk8 : Product  Inputs=*
  cfblk9 : Constant  Value=[390858413.667350]  SampleTime=1
  cfblk2 : Outport
  wires:
  cfblk6/1 -> cfblk12/1(cfblk1)
  cfblk1/1 -> cfblk13/1(cfblk1)
  cfblk11/1(cfblk2) -> cfblk3/1
  cfblk3/1 -> cfblk6/1
  cfblk4/1 -> cfblk2/1
  cfblk16/1 -> cfblk6/2
  cfblk12/1(cfblk2) -> cfblk7/1
  cfblk8/1 -> cfblk10/1(cfblk1)
  cfblk5/1 -> cfblk4/1
  cfblk9/1 -> cfblk11/1(cfblk1)
  cfblk15/1 -> cfblk5/1
  cfblk10/1(cfblk2) -> cfblk17/1
  cfblk17/1 -> cfblk8/1

== system sampleModel26/cfblk154/cfblk19 ==
  cfblk1 : Inport
  cfblk9 : Inport  Port=2
  Action Port : ActionPort  ActionType=else
  cfblk3 : DiscreteIntegrator  SampleTime=-1  ICPrevOutput=DiscIntNeverNeededParam  ICPrevScaledInput=DiscIntNeverNeededParam
  cfblk4 : Math  Operator=pow  SaturateOnIntegerOverflow=on
  cfblk5 : ComplexToMagnitudeAngle
  cfblk6 : Constant  Value=[370127608.905194]  SampleTime=1
  cfblk7 : Subsystem
  cfblk8 : Subsystem
  cfblk2 : Outport
  wires:
  cfblk9/1 -> cfblk7/1(cfblk1)
  cfblk5/1 -> cfblk4/1
  cfblk1/1 -> cfblk8/1(cfblk1)
  cfblk6/1 -> cfblk2/1
  cfblk8/1(cfblk2) -> cfblk5/1
  cfblk5/2 -> cfblk4/2
  cfblk4/1 -> cfblk3/1

== system sampleModel26/cfblk154/cfblk9 ==
  cfblk1 : Inport
  cfblk2 : Outport
  wires:
  cfblk1/1 -> cfblk2/1

== system sampleModel26/cfblk155/cfblk14 ==
  cfblk1 : Inport
  cfblk14 : Inport  Port=2
  cfblk15 : Inport  Port=3
  cfblk16 : Inport  Port=4
  Action Port : ActionPort  ActionType=then
  cfblk10 : Subsystem
  cfblk11 : Subsystem
  cfblk12 : Subsystem
  cfblk13 : Subsystem
  cfblk3 : Delay
  cfblk4 : DiscreteIntegrator  SampleTime=-1  ICPrevOutput=DiscIntNeverNeededParam  ICPrevScaledInput=DiscIntNeverNeededParam
  cfblk5 : MinMax  Inputs=2
  cfblk6 : PermuteDimensions
  cfblk7 : Reshape
  cfblk8 : Gain  Gain=[829221392.636539]
  cfblk9 : Subsystem
  cfblk2 : Outport
  cfblk17 : Outport  Port=2
  wires:
  cfblk5/1 -> cfblk17/1
  cfblk4/1 -> cfblk10/1(cfblk1)
  cfblk8/1 -> cfblk9/1(cfblk1)
  cfblk12/1(cfblk2) -> cfblk11/1(cfblk1)
  cfblk13/1(cfblk2) -> cfblk5/1
  cfblk6/1 -> cfblk12/1(cfblk1)
  cfblk3/1 -> cfblk13/1(cfblk1)
  cfblk16/1 -> cfblk6/1
  cfblk10/1(cfblk2) -> cfblk8/1
  cfblk7/1 -> cfblk5/2
  cfblk15/1 -> cfblk4/1
  cfblk11/1(cfblk2) -> cfblk2/1
  cfblk9/1(cfblk2) -> cfblk3/1
  cfblk14/1 -> cfblk7/1

== system sampleModel26/cfblk155/cfblk15 ==
  cfblk1 : Inport
  cfblk8 : Inport  Port=2
  Action Port : ActionPort  ActionType=else
  cfblk3 : simulink/Discrete/Tapped Delay  vinit=0.0  samptime=-1  NumDelays=1  DelayOrder=Oldest  includeCurrent=off
  cfblk4 : Abs
  cfblk5 : Abs
  cfblk6 : simulink/Math Operations/MinMax Running Resettable  Function=min  vinit=0.0
  cfblk7 : Subsystem
  cfblk9 : Delay
  cfblk2 : Outport
  wires:
  cfblk6/1 -> cfblk3/1
  cfblk8/1 -> cfblk5/1
  cfblk3/1 -> cfblk4/1
  cfblk1/1 -> cfblk6/1
  cfblk5/1 -> cfblk7/1(cfblk1)
  cfblk7/1(cfblk2) -> cfblk2/1
  cfblk4/1 -> cfblk9/1
  cfblk9/1 -> cfblk6/2

== system sampleModel26/cfblk155/cfblk7 ==
  cfblk1 : Inport
  cfblk2 : Outport
  wires:
  cfblk1/1 -> cfblk2/1

== system sampleModel26/cfblk155/cfblk8 ==
  cfblk1 : Inport
  cfblk2 : Outport
  wires:
  cfblk1/1 -> cfblk2/1

== system sampleModel26/cfblk155/cfblk9 ==
  cfblk1 : Inport
  cfblk2 : Outport
  wires:
  cfblk1/1 -> cfblk2/1

== system sampleModel26/cfblk156/cfblk10 ==
  cfblk1 : Inport
  cfblk2 : Outport
  wires:
  cfblk1/1 -> cfblk2/1

== system sampleModel26/cfblk156/cfblk11 ==
  cfblk1 : Inport
  cfblk2 : Outport
  wires:
  cfblk1/1 -> cfblk2/1

== system sampleModel26/cfblk156/cfblk12 ==
  cfblk1 : Inport
  cfblk2 : Outport
  wires:
  cfblk1/1 -> cfblk2/1

== system sampleModel26/cfblk156/cfblk8 ==
  cfblk1 : Inport
  cfblk2 : Outport
  wires:
  cfblk1/1 -> cfblk2/1

== system sampleModel26/cfblk156/cfblk9 ==
  cfblk1 : Inport
  cfblk2 : Outport
  wires:
  cfblk1/1 -> cfblk2/1

== system sampleModel26/cfblk157/cfblk10 ==
  cfblk1 : Inport
  cfblk2 : Outport
  wires:
  cfblk1/1 -> cfblk2/1

== system sampleModel26/cfblk157/cfblk11 ==
  cfblk1 : Inport
  cfblk2 : Outport
  wires:
  cfblk1/1 -> cfblk2/1

== system sampleModel26/cfblk157/cfblk12 ==
  cfblk1 : Inport
  cfblk2 : Outport
  wires:
  cfblk1/1 -> cfblk2/1

== system sampleModel26/cfblk157/cfblk13 ==
  cfblk1 : Inport
  cfblk2 : Outport
  wires:
  cfblk1/1 -> cfblk2/1

== system sampleModel26/cfblk157/cfblk14 ==
  cfblk1 : Inport
  cfblk2 : Outport
  wires:
  cfblk1/1 -> cfblk2/1

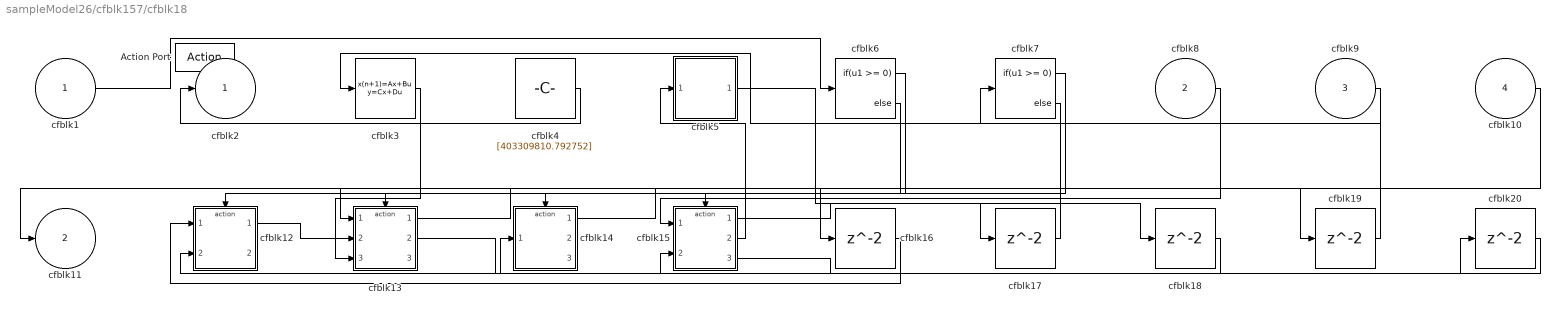
== system sampleModel26/cfblk157/cfblk18 ==
  cfblk1 : Inport
  cfblk8 : Inport  Port=2
  cfblk9 : Inport  Port=3
  cfblk10 : Inport  Port=4
  Action Port : ActionPort  ActionType=then
  cfblk12 : Subsystem  TreatAsAtomicUnit=on
  cfblk13 : Subsystem  TreatAsAtomicUnit=on
  cfblk14 : Subsystem  TreatAsAtomicUnit=on
  cfblk15 : Subsystem  TreatAsAtomicUnit=on
  cfblk{16..20} (5 alike) : Delay
  cfblk3 : DiscreteStateSpace  SampleTime=-1
  cfblk4 : Constant  Value=[403309810.792752]  SampleTime=1
  cfblk5 : Subsystem
  cfblk6 : If  IfExpression=u1 >= 0  SampleTime=1
  cfblk7 : If  IfExpression=u1 >= 0  SampleTime=1
  cfblk2 : Outport
  cfblk11 : Outport  Port=2
  wires:
  cfblk4/1 -> cfblk2/1
  cfblk10/1 -> cfblk11/1
  cfblk1/1 -> cfblk6/1
  cfblk15/2(cfblk14) -> cfblk5/1(cfblk1)
  cfblk12/1(cfblk2) -> cfblk13/2(cfblk9)
  cfblk9/1 -> cfblk3/1
  cfblk3/1 -> cfblk13/3(cfblk10)
  cfblk8/1 -> cfblk15/1(cfblk1)
  cfblk13/2(cfblk11) -> cfblk15/2(cfblk13)
  cfblk6/1 -> cfblk12/Action
  cfblk6/2 -> cfblk13/Action
  cfblk7/1 -> cfblk14/Action
  cfblk7/2 -> cfblk15/Action
  cfblk13/1(cfblk2) -> cfblk16/1
  cfblk16/1 -> cfblk12/1(cfblk1)
  cfblk15/1(cfblk2) -> cfblk17/1
  cfblk17/1 -> cfblk13/1(cfblk1)
  cfblk5/1(cfblk2) -> cfblk18/1
  cfblk18/1 -> cfblk14/1(cfblk1)
  cfblk14/1(cfblk2) -> cfblk19/1
  cfblk19/1 -> cfblk7/1
  cfblk15/3(cfblk15) -> cfblk20/1
  cfblk20/1 -> cfblk12/2(cfblk11)

== system sampleModel26/cfblk157/cfblk19 ==
  cfblk1 : Inport
  cfblk7 : Inport  Port=2
  Action Port : ActionPort  ActionType=else
  cfblk10 : Delay
  cfblk11 : Delay
  cfblk12 : Delay
  cfblk3 : simulink/Discrete/Difference  ICPrevInput=0.0  OutMin=[]  OutMax=[]  OutDataTypeStr=Inherit: Inherit via back propagation  OutDataType=fixdt(1, 16)  OutScaling=2^-10  DoSatur=off
  cfblk4 : DiscreteZeroPole  Poles=[0 0.5]  Gain=1  SampleTime=-1
  cfblk5 : simulink/Math Operations/Slider Gain  gain=1  low=0  high=2
  cfblk6 : If  IfExpression=u1 >= 0  SampleTime=1
  cfblk8 : Subsystem  TreatAsAtomicUnit=on
  cfblk9 : Subsystem  TreatAsAtomicUnit=on
  cfblk2 : Outport
  wires:
  cfblk3/1 -> cfblk6/1
  cfblk1/1 -> cfblk2/1
  cfblk8/1(cfblk2) -> cfblk9/1(cfblk1)
  cfblk4/1 -> cfblk5/1
  cfblk7/1 -> cfblk8/2(cfblk11)
  cfblk8/2(cfblk12) -> cfblk9/2(cfblk14), cfblk9/3(cfblk15)
  cfblk6/1 -> cfblk8/Action
  cfblk6/2 -> cfblk9/Action
  cfblk9/1(cfblk2) -> cfblk10/1
  cfblk10/1 -> cfblk8/1(cfblk1)
  cfblk9/2(cfblk16) -> cfblk11/1
  cfblk11/1 -> cfblk3/1
  cfblk5/1 -> cfblk12/1
  cfblk12/1 -> cfblk4/1

== system sampleModel26/cfblk157/cfblk7 ==
  cfblk1 : Inport
  cfblk2 : Outport
  wires:
  cfblk1/1 -> cfblk2/1

== system sampleModel26/cfblk157/cfblk8 ==
  cfblk1 : Inport
  cfblk2 : Outport
  wires:
  cfblk1/1 -> cfblk2/1

== system sampleModel26/cfblk157/cfblk9 ==
  cfblk1 : Inport
  cfblk2 : Outport
  wires:
  cfblk1/1 -> cfblk2/1

== system sampleModel26/cfblk158/cfblk11 ==
  cfblk1 : Inport
  cfblk2 : Outport
  wires:
  cfblk1/1 -> cfblk2/1

== system sampleModel26/cfblk158/cfblk12 ==
  cfblk1 : Inport
  cfblk2 : Outport
  wires:
  cfblk1/1 -> cfblk2/1

== system sampleModel26/cfblk159/cfblk7 ==
  cfblk1 : Inport
  cfblk2 : Outport
  wires:
  cfblk1/1 -> cfblk2/1

== system sampleModel26/cfblk159/cfblk8 ==
  cfblk1 : Inport
  cfblk2 : Outport
  wires:
  cfblk1/1 -> cfblk2/1

== system sampleModel26/cfblk160/cfblk11 ==
  cfblk1 : Inport
  cfblk2 : Outport
  wires:
  cfblk1/1 -> cfblk2/1

== system sampleModel26/cfblk160/cfblk12 ==
  cfblk1 : Inport
  cfblk2 : Outport
  wires:
  cfblk1/1 -> cfblk2/1

== system sampleModel26/cfblk160/cfblk13 ==
  cfblk1 : Inport
  cfblk2 : Outport
  wires:
  cfblk1/1 -> cfblk2/1

== system sampleModel26/cfblk160/cfblk17 ==
  cfblk1 : Inport
  cfblk12 : Inport  Port=2
  Action Port : ActionPort  ActionType=then
  cfblk10 : Constant  Value=[628162644.706156]  SampleTime=1
  cfblk11 : Subsystem
  cfblk3 : simulink/Discrete/Tapped Delay  vinit=0.0  samptime=-1  NumDelays=1  DelayOrder=Oldest  includeCurrent=off
  cfblk4 : DiscreteFilter
  cfblk5 : PermuteDimensions
  cfblk6 : simulink/Math Operations/Slider Gain  gain=1  low=0  high=2
  cfblk7 : Squeeze
  cfblk8 : Polyval  Coefs=[ +2.081618890e-019, -1.441693666e-014, +4.719686976e-010, -8.536869453e-006, +1.621573104e-001, -8.087801117e+001 ]
  cfblk9 : Constant  Value=[515864445.530394]  SampleTime=1
  cfblk2 : Outport
  wires:
  cfblk5/1 -> cfblk8/1
  cfblk12/1 -> cfblk6/1
  cfblk7/1 -> cfblk11/1(cfblk1)
  cfblk6/1 -> cfblk5/1
  cfblk3/1 -> cfblk2/1
  cfblk11/1(cfblk2) -> cfblk3/1
  cfblk10/1 -> cfblk4/1
  cfblk4/1 -> cfblk7/1

== system sampleModel26/cfblk160/cfblk18 ==
  cfblk1 : Inport
  cfblk10 : Inport  Port=2
  cfblk11 : Inport  Port=3
  Action Port : ActionPort  ActionType=else
  cfblk12 : Delay
  cfblk3 : Sum  Inputs=+
  cfblk4 : Sum  Inputs=+
  cfblk5 : Reshape
  cfblk6 : Subsystem
  cfblk7 : Subsystem
  cfblk8 : Subsystem
  cfblk9 : Subsystem
  cfblk2 : Outport
  wires:
  cfblk11/1 -> cfblk7/1(cfblk1)
  cfblk10/1 -> cfblk6/1(cfblk1)
  cfblk4/1 -> cfblk5/1
  cfblk3/1 -> cfblk8/1(cfblk1)
  cfblk6/1(cfblk2) -> cfblk9/1(cfblk1)
  cfblk8/1(cfblk2) -> cfblk2/1
  cfblk9/1(cfblk2) -> cfblk3/1
  cfblk5/1 -> cfblk12/1
  cfblk12/1 -> cfblk4/1

== system sampleModel26/cfblk161/cfblk10 ==
  cfblk1 : Inport
  cfblk2 : Outport
  wires:
  cfblk1/1 -> cfblk2/1

== system sampleModel26/cfblk161/cfblk11 ==
  cfblk1 : Inport
  cfblk2 : Outport
  wires:
  cfblk1/1 -> cfblk2/1

== system sampleModel26/cfblk161/cfblk12 ==
  cfblk1 : Inport
  cfblk2 : Outport
  wires:
  cfblk1/1 -> cfblk2/1

== system sampleModel26/cfblk161/cfblk13 ==
  cfblk1 : Inport
  cfblk2 : Outport
  wires:
  cfblk1/1 -> cfblk2/1

== system sampleModel26/cfblk161/cfblk8 ==
  cfblk1 : Inport
  cfblk2 : Outport
  wires:
  cfblk1/1 -> cfblk2/1

== system sampleModel26/cfblk161/cfblk9 ==
  cfblk1 : Inport
  cfblk2 : Outport
  wires:
  cfblk1/1 -> cfblk2/1

== system sampleModel26/cfblk154/cfblk18/cfblk10 ==
  cfblk1 : Inport
  cfblk2 : Outport
  wires:
  cfblk1/1 -> cfblk2/1

== system sampleModel26/cfblk154/cfblk18/cfblk11 ==
  cfblk1 : Inport
  cfblk2 : Outport
  wires:
  cfblk1/1 -> cfblk2/1

== system sampleModel26/cfblk154/cfblk18/cfblk12 ==
  cfblk1 : Inport
  cfblk2 : Outport
  wires:
  cfblk1/1 -> cfblk2/1

== system sampleModel26/cfblk154/cfblk18/cfblk13 ==
  cfblk1 : Inport
  cfblk2 : Outport
  wires:
  cfblk1/1 -> cfblk2/1

== system sampleModel26/cfblk154/cfblk19/cfblk7 ==
  cfblk1 : Inport
  cfblk2 : Outport
  wires:
  cfblk1/1 -> cfblk2/1

== system sampleModel26/cfblk154/cfblk19/cfblk8 ==
  cfblk1 : Inport
  cfblk2 : Outport
  wires:
  cfblk1/1 -> cfblk2/1

== system sampleModel26/cfblk155/cfblk14/cfblk10 ==
  cfblk1 : Inport
  cfblk2 : Outport
  wires:
  cfblk1/1 -> cfblk2/1

== system sampleModel26/cfblk155/cfblk14/cfblk11 ==
  cfblk1 : Inport
  cfblk2 : Outport
  wires:
  cfblk1/1 -> cfblk2/1

== system sampleModel26/cfblk155/cfblk14/cfblk12 ==
  cfblk1 : Inport
  cfblk2 : Outport
  wires:
  cfblk1/1 -> cfblk2/1

== system sampleModel26/cfblk155/cfblk14/cfblk13 ==
  cfblk1 : Inport
  cfblk2 : Outport
  wires:
  cfblk1/1 -> cfblk2/1

== system sampleModel26/cfblk155/cfblk14/cfblk9 ==
  cfblk1 : Inport
  cfblk2 : Outport
  wires:
  cfblk1/1 -> cfblk2/1

== system sampleModel26/cfblk155/cfblk15/cfblk7 ==
  cfblk1 : Inport
  cfblk2 : Outport
  wires:
  cfblk1/1 -> cfblk2/1

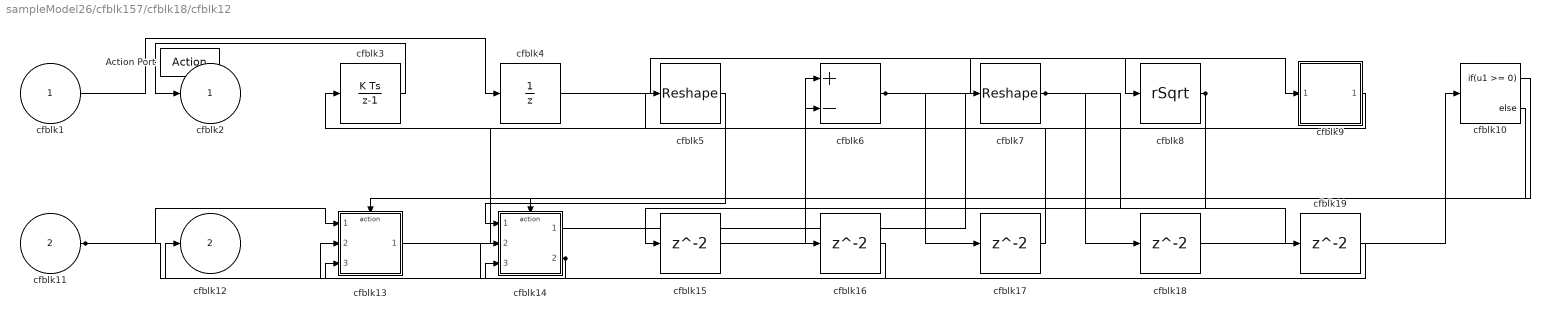
== system sampleModel26/cfblk157/cfblk18/cfblk12 ==
  cfblk1 : Inport
  cfblk11 : Inport  Port=2
  Action Port : ActionPort  ActionType=then
  cfblk10 : If  IfExpression=u1 >= 0  SampleTime=1
  cfblk13 : Subsystem  TreatAsAtomicUnit=on
  cfblk14 : Subsystem  TreatAsAtomicUnit=on
  cfblk{15..19} (5 alike) : Delay
  cfblk3 : DiscreteIntegrator  SampleTime=-1  ICPrevOutput=DiscIntNeverNeededParam  ICPrevScaledInput=DiscIntNeverNeededParam
  cfblk4 : UnitDelay  SampleTime=-1
  cfblk5 : Reshape
  cfblk6 : Sum  Inputs=+-
  cfblk7 : Reshape
  cfblk8 : Sqrt  Operator=rSqrt  AlgorithmType=Newton-Raphson  SaturateOnIntegerOverflow=on
  cfblk9 : Subsystem
  cfblk2 : Outport
  cfblk12 : Outport  Port=2
  wires:
  cfblk7/1 -> cfblk18/1, cfblk19/1
  cfblk6/1 -> cfblk8/1, cfblk17/1
  cfblk9/1(cfblk2) -> cfblk3/1
  cfblk13/1(cfblk2) -> cfblk6/1
  cfblk14/1(cfblk2) -> cfblk7/1
  cfblk3/1 -> cfblk2/1
  cfblk4/1 -> cfblk9/1(cfblk1)
  cfblk8/1 -> cfblk15/1, cfblk16/1
  cfblk5/1 -> cfblk14/1(cfblk1)
  cfblk1/1 -> cfblk4/1
  cfblk14/2(cfblk16) -> cfblk12/1, cfblk13/3(cfblk13)
  cfblk11/1 -> cfblk13/1(cfblk1), cfblk14/3(cfblk15)
  cfblk10/1 -> cfblk13/Action
  cfblk10/2 -> cfblk14/Action
  cfblk15/1 -> cfblk6/2
  cfblk16/1 -> cfblk14/2(cfblk14)
  cfblk17/1 -> cfblk5/1
  cfblk18/1 -> cfblk10/1
  cfblk19/1 -> cfblk13/2(cfblk12)

== system sampleModel26/cfblk157/cfblk18/cfblk13 ==
  cfblk1 : Inport
  cfblk9 : Inport  Port=2
  cfblk10 : Inport  Port=3
  Action Port : ActionPort  ActionType=else
  cfblk13 : Delay
  cfblk3 : DiscreteTransferFcn
  cfblk4 : DotProduct  InputSameDT=on  OutDataTypeStr=Inherit: Inherit via internal rule
  cfblk5 : Sum  Inputs=|++
  cfblk6 : Signum
  cfblk7 : DotProduct  InputSameDT=on  OutDataTypeStr=Inherit: Inherit via internal rule
  cfblk8 : Subsystem
  cfblk2 : Outport
  cfblk11 : Outport  Port=2
  cfblk12 : Outport  Port=3
  wires:
  cfblk8/1(cfblk2) -> cfblk7/1, cfblk5/2
  cfblk9/1 -> cfblk2/1
  cfblk3/1 -> cfblk7/2
  cfblk1/1 -> cfblk6/1
  cfblk7/1 -> cfblk4/1
  cfblk10/1 -> cfblk8/1(cfblk1)
  cfblk6/1 -> cfblk3/1, cfblk11/1, cfblk12/1
  cfblk4/1 -> cfblk5/1
  cfblk5/1 -> cfblk13/1
  cfblk13/1 -> cfblk4/2

== system sampleModel26/cfblk157/cfblk18/cfblk14 ==
  cfblk1 : Inport
  Action Port : ActionPort  ActionType=then
  cfblk3 : UnaryMinus
  cfblk4 : Subsystem
  cfblk5 : Subsystem
  cfblk6 : Subsystem
  cfblk2 : Outport
  cfblk7 : Outport  Port=2
  cfblk8 : Outport  Port=3
  wires:
  cfblk3/1 -> cfblk7/1, cfblk2/1
  cfblk4/1(cfblk2) -> cfblk8/1
  cfblk6/1(cfblk2) -> cfblk5/1(cfblk1), cfblk4/1(cfblk1)
  cfblk5/1(cfblk2) -> cfblk3/1
  cfblk1/1 -> cfblk6/1(cfblk1)
